simulink model "Sim"  (R2017a)
settings: Solver=VariableStepAuto  StartTime=0.0  StopTime=10.0  MinStep=0.001  RelTol=1e-3
values from neighbouring files (symbols this model uses):
  C = [1 0 0 0 0 0 ... (first row only)    [Data.m]
  X0 = [-1 1 1 1 1 1]'*0.1    [Data.m]
settings Model: Creator=pblaud2017  LastModifiedBy=pblaud2017

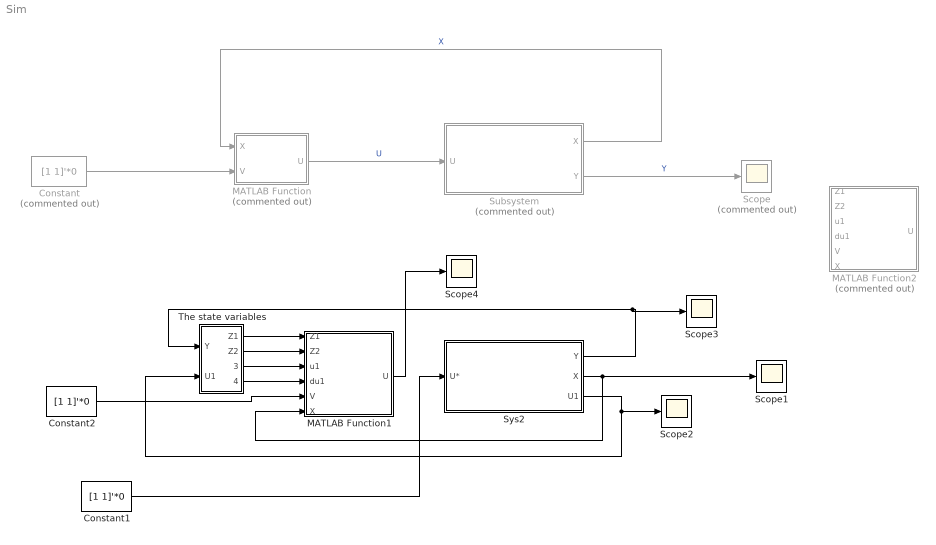
== system Sim ==
  Constant : Constant  Commented=on  Value=[1 1]'*0
  Constant1 : Constant  Value=[1 1]'*0
  Constant2 : Constant  Value=[1 1]'*0
  MATLAB Function : MATLAB Function  Commented=on  TreatAsAtomicUnit=on
  MATLAB Function1 : MATLAB Function  TreatAsAtomicUnit=on
  MATLAB Function2 : MATLAB Function  Commented=on  TreatAsAtomicUnit=on
  Scope : Scope  Commented=on
  Scope{1..4} (4 alike) : Scope
  Subsystem : Subsystem  Commented=on
  Sys2 : Subsystem
  The state variables : Subsystem
  wires:
  Subsystem/2(Y) -> Scope/1  "Y"
  Subsystem/1(X) -> MATLAB Function/1(X)  "X"
  MATLAB Function/1(U) -> Subsystem/1(U)  "U"
  Constant/1 -> MATLAB Function/2(V)
  Sys2/2(X) -> MATLAB Function1/6(X), Scope1/1
  Sys2/3(U1) -> The state variables/2(U1), Scope2/1
  Constant1/1 -> Sys2/1(U*)
  The state variables/1(Z1) -> MATLAB Function1/1(Z1)
  The state variables/2(Z2) -> MATLAB Function1/2(Z2)
  The state variables/3(U1.) -> MATLAB Function1/3(u1)
  The state variables/4(dU1) -> MATLAB Function1/4(du1)
  Sys2/1(Y) -> Scope3/1, The state variables/1(Y)
  Constant2/1 -> MATLAB Function1/5(V)
  MATLAB Function1/1(U) -> Scope4/1

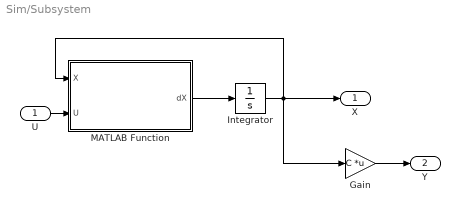
== system Sim/Subsystem ==
  U : Inport
  Gain : Gain  Gain=C  Multiplication=Matrix(K*u) (u vector)
  Integrator : Integrator  InitialCondition=X0
  MATLAB Function : MATLAB Function  TreatAsAtomicUnit=on
  X : Outport
  Y : Outport  Port=2
  wires:
  U/1 -> MATLAB Function/2(U)
  MATLAB Function/1(dX) -> Integrator/1
  Integrator/1 -> Gain/1, X/1, MATLAB Function/1(X)
  Gain/1 -> Y/1

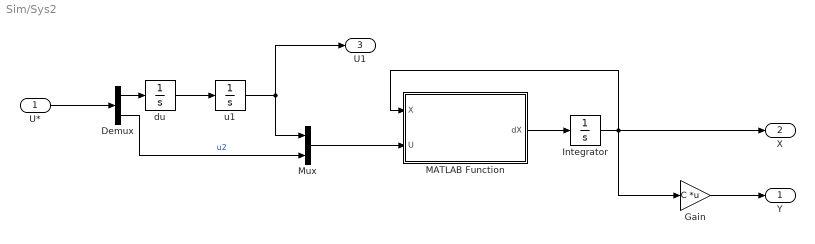
== system Sim/Sys2 ==
  U* : Inport
  Demux : Demux  Outputs=2
  Gain : Gain  Gain=C  Multiplication=Matrix(K*u) (u vector)
  Integrator : Integrator  InitialCondition=X0
  MATLAB Function : MATLAB Function  TreatAsAtomicUnit=on
  Mux : Mux  Inputs=2
  du : Integrator
  u1 : Integrator  InitialCondition=1
  Y : Outport
  X : Outport  Port=2
  U1 : Outport  Port=3
  wires:
  MATLAB Function/1(dX) -> Integrator/1
  Integrator/1 -> Gain/1, X/1, MATLAB Function/1(X)
  Gain/1 -> Y/1
  du/1 -> u1/1
  u1/1 -> U1/1, Mux/1
  Mux/1 -> MATLAB Function/2(U)
  Demux/1 -> du/1
  U*/1 -> Demux/1
  Demux/2 -> Mux/2  "u2"

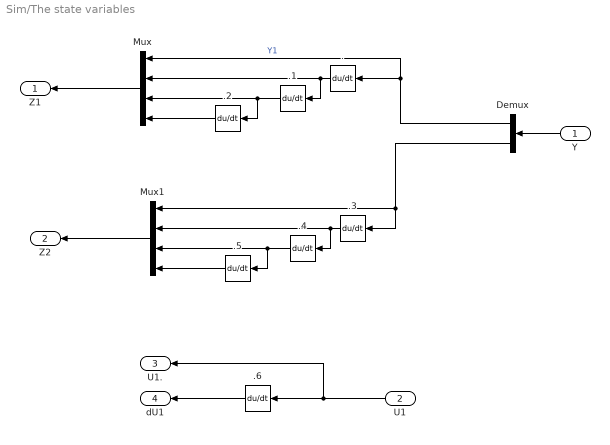
== system Sim/The state variables ==
  Y : Inport
  U1 : Inport  Port=2
  .{,1..6} (7 alike) : Derivative
  Demux : Demux  Outputs=2
  Mux : Mux
  Mux1 : Mux
  Z1 : Outport
  Z2 : Outport  Port=2
  U1. : Outport  Port=3
  dU1 : Outport  Port=4
  wires:
  Demux/1 -> ./1, Mux/1  "Y1"
  ./1 -> .1/1, Mux/2
  .1/1 -> .2/1, Mux/3
  .2/1 -> Mux/4
  Mux/1 -> Z1/1
  Mux1/1 -> Z2/1
  .5/1 -> Mux1/4
  .4/1 -> Mux1/3, .5/1
  .3/1 -> Mux1/2, .4/1
  Demux/2 -> Mux1/1, .3/1
  U1/1 -> U1./1, .6/1
  .6/1 -> dU1/1
  Y/1 -> Demux/1

== matlab function Sim/MATLAB Function ==
  data: X input; V input; U output
function U = fcn(X,V)
e=10^-3;
x1 = X(1);
x2 = X(2);
x3 = X(3);
x4 = X(4);
x5 = X(5);
x6 = X(6);
v1 =V(1);
v2 =V(2);
%% The eigenvalues:
p1 = -2; p2 = -2;
k1 = p1*p2;
k2 = -p1-p2;
k3 = k1;
k4 = k2 ;
w1 = -k1*x1-k2*x2 + v1 ;
w2 = -k3*x1-k4*x2 + v2 ;
W = [w1;w2];
%% Transformation from W to U;
Bu = [-sin(x5)   e*cos(x5)
    cos(x5)   e*sin(x5)];

a = Bu\[0;1];
b = inv(Bu);
U = a + b*W;

== matlab function Sim/Subsystem/MATLAB Function ==
  data: X input; dX output; U input
function dX = fcn(X,U)

e=10^-3;
x1 = X(1);
x2 = X(2);
x3 = X(3);
x4 = X(4);
x5 = X(5);
x6 = X(6);

u1 = U(1);
u2 = U(2);

dX = [x2
    -sin(x5)*u1 + e*cos(x5)*u2
    x4
    cos(x5)*u1 + e*sin(x5)*u2-1
    x6
    u2];

== matlab function Sim/Sys2/MATLAB Function ==
  data: X input; dX output; U input
function dX = fcn(X,U)

e=0;
x1 = X(1);
x2 = X(2);
x3 = X(3);
x4 = X(4);
x5 = X(5);
x6 = X(6);

u1 = U(1);
u2 = U(2);

dX = [x2
    -sin(x5)*u1 + e*cos(x5)*u2
    x4
    cos(x5)*u1 + e*sin(x5)*u2-1
    x6
    u2];

== matlab function Sim/MATLAB Function1 ==
  data: Z1 input; Z2 input; u1 input; du1 input; V input; X input; U output
function U = fcn(Z1,Z2,u1,du1,V,X)


x1 = X(1);
x2 = X(2);
x3 = X(3);
x4 = X(4);
x5 = X(5);
x6 = X(6);
v1 =V(1);
v2 =V(2);

k1=16 ; k2=32; k3= 24; k4=8 ;

y1 = Z1(1) ;
dy1 = Z1(2) ;
ddy1 = Z1(3) ;
dddy1 = Z1(4) ;

y2 = Z2(1) ;
dy2 = Z2(2) ;
ddy2 = Z2(3) ;
dddy2 = Z2(4) ;

%% The eigenvalues:

w1 = -k1*y1-k2*dy1 + k3*ddy1 +k4*dddy1 +v1 ;
w2 = -k1*y2-k2*dy2 + k3*ddy2 +k4*dddy2 +v2 ;
W = [w1;w2];
%% Transformation from W to U;

beta = [-sin(x5) -u1*cos(x5)
        cos(x5)    -u1*sin(x5)];
alpha = [-2*du1*x6*cos(x5)+u1*sin(x5)*x6^2;
         -2*du1*x6*sin(x5)-u1*x6^2*cos(x5)];
       
      
U = beta\W - beta\ alpha;

== matlab function Sim/MATLAB Function2 ==
  data: Z1 input; Z2 input; u1 input; du1 input; V input; X input; U output
function U = fcn(Z1,Z2,u1,du1,V,X)


x1 = X(1);
x2 = X(2);
x3 = X(3);
x4 = X(4);
x5 = X(5);
x6 = X(6);
v1 =V(1);
v2 =V(2);

k1=16 ; k2= 32   ; k3= 24  ; k4=   8 ;

y1 = Z1(1) ;
dy1 = Z1(2) ;
ddy1 = Z1(3) ;
dddy1 = Z1(4) ;

y2 = Z2(1) ;
dy2 = Z2(2) ;
ddy2 = Z2(3) ;
dddy2 = Z2(4) ;

%% The eigenvalues:

w1 = -k1*y1-k2*dy1 + k3*ddy1 +k4*dddy1 +v1 ;
w2 = -k1*y2-k2*dy2 + k3*ddy2 +k4*dddy2 +v2 ;
W = [w1;w2];
%% Transformation from W to U;

beta = [-sin(x5) -u1*cos(x5)
        cos(x5)    -u1*sin(x5)];
alpha = [-2*du1*x6*cos(x5)+u1*sin(x5)*x6^2;
         -2*du1*x6*sin(x5)-u1*x6^2*cos(x5)]
       
      
U = beta\W - beta\ alpha;
